simulink model "Ex5_3_iii_iv"  (R2022b)
settings: Solver=ode4  StartTime=0.0  StopTime=50  FixedStep=0.001  RelTol=1e-3
values from neighbouring files (symbols this model uses):
  par =     [par.mat]
settings Model: Creator=super  LastModifiedBy=15043
settings ModelReferenceCC: EnableRefExpFcnMdlSchedulingChecks=on

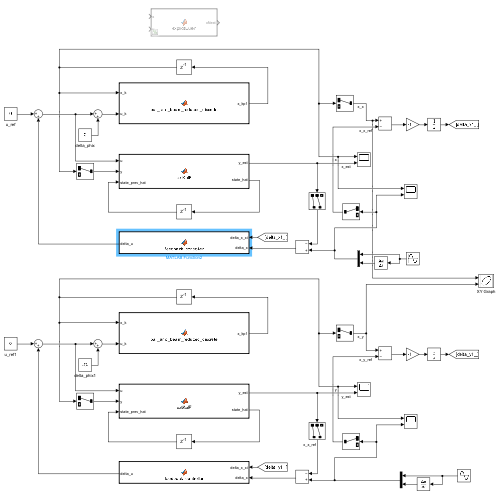
[thumbnail: Simulink's stored preview of the top-level diagram]
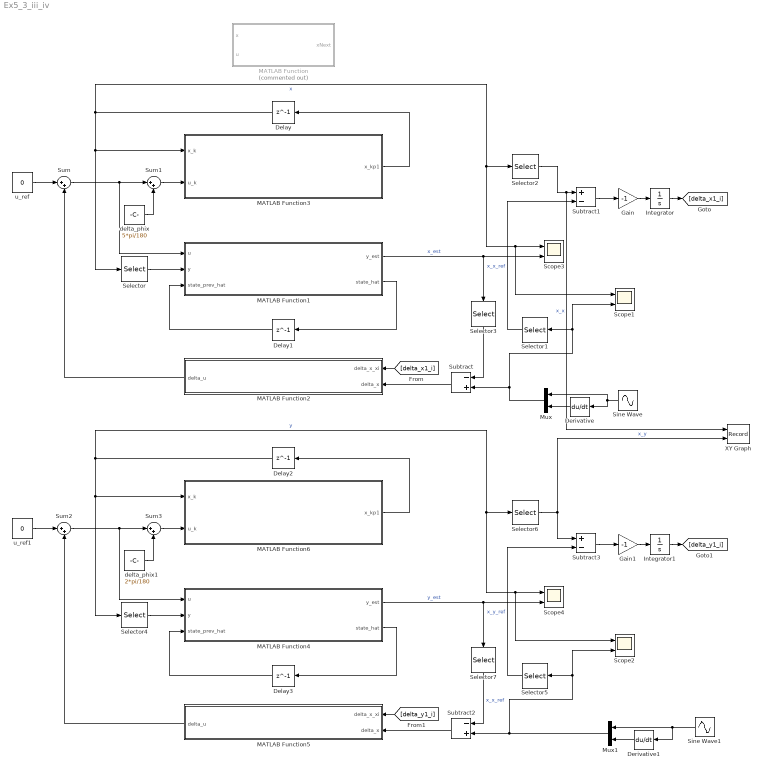
== system Ex5_3_iii_iv ==
  Delay : Delay  DelayLength=1  InitialCondition=par.ex5_7_iii_x0
  Delay1 : Delay  DelayLength=1  InitialCondition=par.ex5_6_iii_x0_hat  UseCircularBuffer=on
  Delay2 : Delay  DelayLength=1  InitialCondition=par.ex5_7_iii_x0
  Delay3 : Delay  DelayLength=1  InitialCondition=par.ex5_6_iii_x0_hat  UseCircularBuffer=on
  Derivative : Derivative
  Derivative1 : Derivative
  Gain : Gain  Gain=-1
  Gain1 : Gain  Gain=-1
  Integrator : Integrator
  Integrator1 : Integrator
  MATLAB Function : MATLAB Function  Commented=on  TreatAsAtomicUnit=on
  MATLAB Function1 : MATLAB Function  TreatAsAtomicUnit=on
  MATLAB Function2 : MATLAB Function  TreatAsAtomicUnit=on
  MATLAB Function3 : MATLAB Function  TreatAsAtomicUnit=on
  MATLAB Function4 : MATLAB Function  TreatAsAtomicUnit=on
  MATLAB Function5 : MATLAB Function  TreatAsAtomicUnit=on
  MATLAB Function6 : MATLAB Function  TreatAsAtomicUnit=on
  Mux : Mux  Inputs=2
  Mux1 : Mux  Inputs=2
  Scope{1..4} (4 alike) : Scope  NumInputPorts=2
  Selector{,1..2,4..6} (6 alike) : Selector  InputPortWidth=2  IndexOptions=Index vector (dialog)  Indices=[1]  OutputSizes=1
  Selector3 : Selector  InputPortWidth=3  IndexOptions=Index vector (dialog)  Indices=[1 2]  OutputSizes=1
  Selector7 : Selector  InputPortWidth=3  IndexOptions=Index vector (dialog)  Indices=[1 2]  OutputSizes=1
  Sine Wave : Sin  Amplitude=par.A_x  Frequency=par.f_x  Phase=par.P_x  SampleTime=0
  Sine Wave1 : Sin  Amplitude=par.A_y  Frequency=par.f_y  Phase=par.P_y  SampleTime=0
  Subtract : Sum  Inputs=-+
  Subtract1 : Sum  Inputs=+-
  Subtract2 : Sum  Inputs=-+
  Subtract3 : Sum  Inputs=+-
  Sum{,1..3} (4 alike) : Sum  Inputs=|++
  XY Graph : Record  FileSettingsInternal="{\"entries\":[{\"content\":{\"excelSettings\":{\"content\":{},\"type\":\"Streamout.ExcelSettings\"}},\"type\":\"Streamout.FileSettingStorage\",\"uuid\":\"a4bbb464-e277-446f-938f-6bfab3576abf\"}],\"packageUris\":[\"http://schema.mathworks.com/mf0/streamout_blocks/R2020a\"],\"version\":\"1.0\"}"  Layout=[1 1]  SignalsInternal="{\"entries\":[{\"content\":{\"signals\":[{\"content\":{\"blockPath\":[\"Ex5_3_iii_iv/XY Graph\"],\"channel\":[],\"dimensions\":[1],\"domain\":\"Ex5_3_iii_iv/XY Graph\",\"lineColor\":\"#fe330a\",\"plots\":[1],\"port\":1,\"sid\":[\"\"],\"signalID\":734,\"signalName\":\"x_x\"},\"type\":\"RecordBlkView.Signal\",\"uuid\":\"eadc8627-04eb-4cba-99ca-edfee08eab61\"},{\"content\":{\"blockPath\":[\"Ex5_3_iii_iv/XY Graph\"],\"channel\":[],\"dimensions\":[1],\"domain\":\"Ex5_3_iii_iv/XY Graph\",\"lineColor\":\"#22b573\",\"plots\":[1],\"port\":2,\"sid\":[\"\"],\"signalID\":738,\"signalName\":\"x_y\"},\"type\":\"RecordBlkView.Signal\",\"uuid\":\"8ab3a3d5-7a29-4cdb-8e64-73b846e4f8a4\"}]},\"type\":\"RecordBlkView.InputSignals\",\"uuid\":\"6970aaac-69ae-4046-88bf-16af4de119b8\"}],\"packageUris\":[\"http://schema.mathworks.com/mf0/streamout_blocks/R2020a\"],\"version\":\"1.0\"}"  VisualizationBindings="{\"xyplotplugin\":{\"info\":[{\"series\":[{\"bindingParametersList\":[{\"parameter\":\"Y-Axis\",\"signalID\":738,\"signalName\":\"x_y\"},{\"parameter\":\"X-Axis\",\"signalID\":734,\"signalName\":\"x_x\"}],\"seriesID\":877}],\"subplotID\":1}]}}"  CompatibilityTag=XY
  delta_phix : Constant  Value=5*pi/180
  delta_phix1 : Constant  Value=2*pi/180
  u_ref : Constant  Value=0
  u_ref1 : Constant  Value=0
  wires:
  Delay/1 -> MATLAB Function3/1(x_k), Selector/1, Scope1/1, Scope3/1, Selector2/1  "x"
  MATLAB Function1/2(state_hat) -> Delay1/1
  Delay1/1 -> MATLAB Function1/3(state_prev_hat)
  Selector/1 -> MATLAB Function1/2(y)
  MATLAB Function1/1(y_est) -> Selector3/1, Scope3/2  "x_est"
  Subtract/1 -> MATLAB Function2/2(delta_x)
  u_ref/1 -> Sum/1
  Sum/1 -> Sum1/1, MATLAB Function1/1(u)
  MATLAB Function3/1(x_kp1) -> Delay/1
  MATLAB Function2/1(delta_u) -> Sum/2
  Mux/1 -> Scope1/2, Selector1/1, Subtract/2
  Sum1/1 -> MATLAB Function3/2(u_k)
  delta_phix/1 -> Sum1/2
  Gain/1 -> Integrator/1
  Subtract1/1 -> Gain/1
  Selector2/1 -> XY Graph/1, Subtract1/1  "x_x"
  Integrator/1 -> [delta_x1_i]
  Selector1/1 -> Subtract1/2  "x_x_ref"
  [delta_x1_i] -> MATLAB Function2/1(delta_x_xi)
  Selector3/1 -> Subtract/1
  Selector5/1 -> Subtract3/2  "x_y_ref"
  [delta_y1_i] -> MATLAB Function5/1(delta_x_xi)
  Selector7/1 -> Subtract2/1  "x_x_ref"
  Selector6/1 -> XY Graph/2, Subtract3/1  "x_y"
  Gain1/1 -> Integrator1/1
  Sum3/1 -> MATLAB Function6/2(u_k)
  Subtract2/1 -> MATLAB Function5/2(delta_x)
  u_ref1/1 -> Sum2/1
  Integrator1/1 -> [delta_y1_i]
  Subtract3/1 -> Gain1/1
  Sum2/1 -> Sum3/1, MATLAB Function4/1(u)
  MATLAB Function6/1(x_kp1) -> Delay2/1
  delta_phix1/1 -> Sum3/2
  MATLAB Function4/1(y_est) -> Selector7/1, Scope4/2  "y_est"
  Mux1/1 -> Scope2/2, Selector5/1, Subtract2/2
  Selector4/1 -> MATLAB Function4/2(y)
  Delay2/1 -> MATLAB Function6/1(x_k), Selector4/1, Scope2/1, Scope4/1, Selector6/1  "y"
  MATLAB Function4/2(state_hat) -> Delay3/1
  MATLAB Function5/1(delta_u) -> Sum2/2
  Delay3/1 -> MATLAB Function4/3(state_prev_hat)
  Sine Wave/1 -> Mux/1, Derivative/1
  Derivative/1 -> Mux/2
  Derivative1/1 -> Mux1/2
  Sine Wave1/1 -> Derivative1/1, Mux1/1

== matlab function Ex5_3_iii_iv/MATLAB Function2 ==
  data: delta_x_xi input; delta_x input; delta_u output; par parameter
function delta_u = feedback_controller(delta_x_xi,delta_x,par)

k = par.ex5_3_iv_k;
ki = 0;
delta_u = k*delta_x + ki*delta_x_xi;

end

== matlab function Ex5_3_iii_iv/MATLAB Function ==
  data: x input; u input; xNext output; par parameter
function xNext = explicitEuler(x,u,par)
 
    h = par.timeStep;
    xNext = x + h*reducedModel( x, u, par);

end

function dx = reducedModel( x, u, par )
    
    % system parameters   
    g = par.g;

    % States vector
    x2 = x(2);

    % Preallocate
    dx = zeros(2,1);

    % reduced model
    dx(1) = x2;
    dx(2) = -(5/7)*g*sin(u);
end

== matlab function Ex5_3_iii_iv/MATLAB Function1 ==
  data: y_est output; u input; state_hat output; y input; state_prev_hat input; par parameter
function [y_est, state_hat] = extKalF(u, y, state_prev_hat, par )
    
    R = par.R;          % Measurement covariance matrix
    Q = par.Q6;          % Process covariance matrix
    g = par.g;

    ts = par.timeStep;  % discretization timestep for the explicit euler

    c = 0.1;
    h = @(x) x(1)+c*x(3);    % As we only measure the first state
    
    H = [1 0 c];          % Measurement Jacobian        
       
    x_hat_prev = state_prev_hat(1:3, :);

    dF = [ 0 1 0; 0 0 -5*g*cos( u + x_hat_prev(3,:) )/7; 0 0 0];   % State jacobian 

    P_prev = reshape( state_prev_hat(4:end), 3,3);
    
    % discretize the nonlinear model
    fd = x_hat_prev + ts*f( x_hat_prev, u, par );
    
    % discretize the jacobian
    F = eye(3) + ts*dF;

    %%%%%% Predict step %%%%%%
    x_hatm = fd;
    Pm = F*P_prev*F' + Q;
    
    %%%%%% Update step %%%%%%
    K = Pm*H'/((H*Pm*H'+ R));         % Kalman gain
    
    x_hat = x_hatm + K*(y-h(x_hatm));   
    P = ( eye(3) - K*H)*Pm ;
         
    state_hat = [x_hat; P(:);];
    y_est = x_hat_prev;
 end


function dx = f( x, u, par )
    
    % system parameters   
    g = par.g;

    % States vector
    x2 = x(2);
    x3 = x(3);

    % Preallocate
    dx = zeros(3,1);

    % reduced model
    dx(1) = x2;
    dx(2) = -(5/7)*g*sin(u+x3);
    dx(3) = 0;
end

== matlab function Ex5_3_iii_iv/MATLAB Function3 ==
  data: x_k input; u_k input; x_kp1 output; par parameter
function x_kp1 = ball_and_beam_reduced_discrete(x_k, u_k, par)
%#codegen
x_kp1 = ball_and_beam_reduced_discrete(x_k, u_k, par);

== matlab function Ex5_3_iii_iv/MATLAB Function4 ==
  data: y_est output; u input; state_hat output; y input; state_prev_hat input; par parameter
function [y_est, state_hat] = extKalF(u, y, state_prev_hat, par )
    
    R = par.R;          % Measurement covariance matrix
    Q = par.Q6;          % Process covariance matrix
    g = par.g;

    ts = par.timeStep;  % discretization timestep for the explicit euler

    c = 0.1;
    h = @(x) x(1)+c*x(3);    % As we only measure the first state
    
    H = [1 0 c];          % Measurement Jacobian        
       
    x_hat_prev = state_prev_hat(1:3, :);

    dF = [ 0 1 0; 0 0 -5*g*cos( u + x_hat_prev(3,:) )/7; 0 0 0];   % State jacobian 

    P_prev = reshape( state_prev_hat(4:end), 3,3);
    
    % discretize the nonlinear model
    fd = x_hat_prev + ts*f( x_hat_prev, u, par );
    
    % discretize the jacobian
    F = eye(3) + ts*dF;

    %%%%%% Predict step %%%%%%
    x_hatm = fd;
    Pm = F*P_prev*F' + Q;
    
    %%%%%% Update step %%%%%%
    K = Pm*H'/((H*Pm*H'+ R));         % Kalman gain
    
    x_hat = x_hatm + K*(y-h(x_hatm));   
    P = ( eye(3) - K*H)*Pm ;
         
    state_hat = [x_hat; P(:);];
    y_est = x_hat_prev;
 end


function dx = f( x, u, par )
    
    % system parameters   
    g = par.g;

    % States vector
    x2 = x(2);
    x3 = x(3);

    % Preallocate
    dx = zeros(3,1);

    % reduced model
    dx(1) = x2;
    dx(2) = -(5/7)*g*sin(u+x3);
    dx(3) = 0;
end

== matlab function Ex5_3_iii_iv/MATLAB Function5 ==
  data: delta_x_xi input; delta_x input; delta_u output; par parameter
function delta_u = feedback_controller(delta_x_xi,delta_x,par)

k = par.ex5_3_iv_k;
ki = -2;
delta_u = k*delta_x + ki*delta_x_xi;

end

== matlab function Ex5_3_iii_iv/MATLAB Function6 ==
  data: x_k input; u_k input; x_kp1 output; par parameter
function x_kp1 = ball_and_beam_reduced_discrete(x_k, u_k, par)
%#codegen
x_kp1 = ball_and_beam_reduced_discrete(x_k, u_k, par);
